simulink model "No5_QuadcopterAltitudeControl"  (R2022a)
settings: Solver=FixedStepDiscrete  StartTime=0.0  StopTime=inf  RelTol=1e-3  EnableMultiTasking=on
undefined symbols (not defined in the file): dev, DiscIntNeverNeededParam, Main, pwm_output0
libraries: simulink x1, px4lib x1, px4uORBlib x1
settings Model: ExtModeTrigDuration=10  Creator=liuwhale  LastModifiedBy=liuwhale
settings SolverCC: PositivePriorityOrder=on
settings OptimizationCC: EnhancedBackFolding=on  PassReuseOutputArgsAs=Individual arguments  ZeroExternalMemoryAtStartup=off  ZeroInternalMemoryAtStartup=off  MaxStackSize=64  OptimizeBlockOrder=speed  DifferentSizesBufferReuse=on  OptimizationCustomize=off  EfficientTunableParamExpr=on
settings DebuggingCC: ParameterTunabilityLossMsg=error
settings HardwareCC: ProdBitPerPointer=32  ProdBitPerSizeT=32  ProdBitPerPtrDiffT=32  ProdLargestAtomicInteger=Long  ProdLargestAtomicFloat=Double  ProdWordSize=32  ProdLongLongMode=on  ProdHWDeviceType=ARM Compatible->ARM Cortex
settings SFSimCC: MATLABDynamicMemAlloc=off  SimTargetLang=C++
settings RTWCC: SystemTargetFile=ert.tlc  HardwareBoard=PX4 Host Target  TLCOptions="-aInlineSetEventsForThisBaseRateFcn=TLC_FALSE -aSuppressMultiTaskScheduler=TLC_FALSE  -aRateBasedStepFcn=0"  TemplateMakefile=ert_default_tmf  Toolchain=GNU Tools for PX4 Autopilots  PortableWordSizes=on  TargetLang=C++
settings CodeAppCC: ForceParamTrailComments=on  IgnoreCustomStorageClasses=off  OperatorAnnotations=on  SimulinkDataObjDesc=on  SFDataObjDesc=on  InsertBlockDesc=on
settings ERTTargetCC: ExtModeStaticAlloc=on

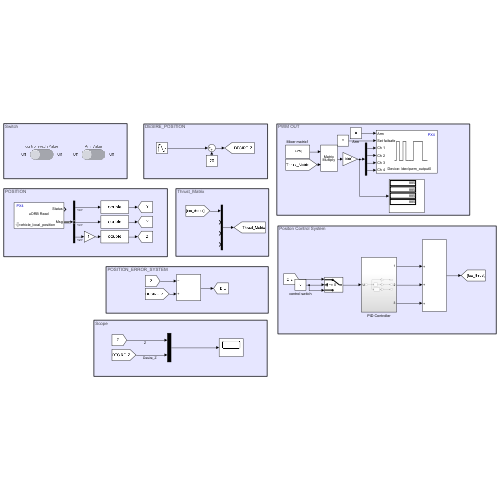
[thumbnail: Simulink's stored preview of the top-level diagram]
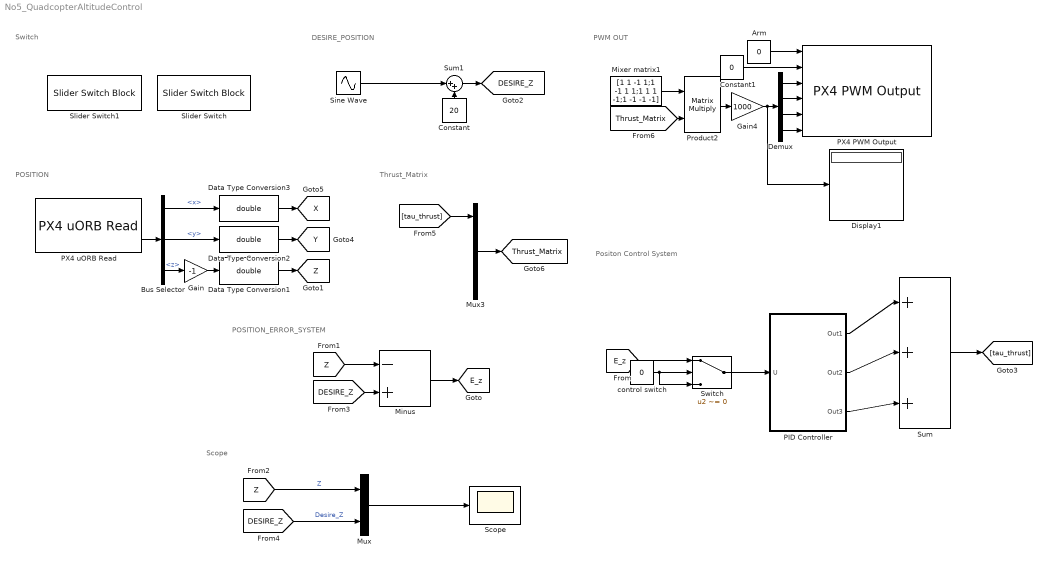
== system No5_QuadcopterAltitudeControl ==
  note: PWM OUT
  note: Scope
  note: Positon Control System
  note: Thrust_Matrix
  note: POSITION_ERROR_SYSTEM
  note: POSITION
  note: DESIRE_POSITION
  note: Switch
  Arm : Constant  Value=0  OutDataTypeStr=boolean
  Bus Selector : BusSelector  OutputSignals=x,y,z
  Constant : Constant  Value=20
  Constant1 : Constant  Value=0  OutDataTypeStr=boolean
  Data Type Conversion1 : DataTypeConversion  OutDataTypeStr=double  SaturateOnIntegerOverflow=off  RndMeth=Floor
  Data Type Conversion2 : DataTypeConversion  OutDataTypeStr=double  SaturateOnIntegerOverflow=off  RndMeth=Floor
  Data Type Conversion3 : DataTypeConversion  OutDataTypeStr=double  SaturateOnIntegerOverflow=off  RndMeth=Floor
  Demux : Demux
  Display1 : Display
  Gain : Gain  Gain=-1
  Gain4 : Gain  Gain=1000  OutDataTypeStr=uint16
  Minus : Sum  Inputs=-+
  Mixer matrix1 : Constant  Value=[1 1 -1 1;1 -1 1 1;1 1 1 -1;1 -1 -1 -1]  OutDataTypeStr=Inherit: Inherit via back propagation
  Mux : Mux  Inputs=2
  Mux3 : Mux
  PID Controller : Subsystem
  PX4 PWM Output : px4lib/PX4 PWM Output  pwmDevice=Main (/dev/pwm_output0)  pwmChannel1_=on  pwmChannel2_=on  pwmChannel3_=on  pwmChannel4_=on  pwmChannel5_=off  pwmChannel6_=off  pwmChannel7_=off  pwmChannel8_=off  forceTerminateFailsafe=off  outputErrorStatus=off
      settings: SourceProductBaseCode=PX4AUTOPILOTS
  PX4 uORB Read : px4uORBlib/PX4 uORB Read  uORBTopic=vehicle_local_position  selectInstance=vehicle_local_position  SampleTime=0.001  BlockingMode=off  BlockTimeout=1e-3
      settings: SourceProductBaseCode=PX4AUTOPILOTS
  Product2 : Product  Multiplication=Matrix(*)  RndMeth=Zero
  Scope : Scope
  Sine Wave : Sin  Amplitude=20  SampleTime=0
  Slider Switch : SliderSwitchBlock
      settings: Values={{'Off', 'On'}, [0 1]}
  Slider Switch1 : SliderSwitchBlock
      settings: Values={{'Off', 'On'}, [0 1]}
  Sum : Sum  Inputs=|+++
  Sum1 : Sum  Inputs=|++
  Switch : Switch  Criteria=u2 ~= 0  SaturateOnIntegerOverflow=off  InputSameDT=off
  control switch : Constant  Value=0
  tag scope: DESIRE_Z=global, E_z=global, Thrust_Matrix=global, X=global, Y=global, Z=global
  wires:
  Arm/1 -> PX4 PWM Output/1
  Constant1/1 -> PX4 PWM Output/2
  Mixer matrix1/1 -> Product2/1
  Product2/1 -> Gain4/1
  Demux/1 -> PX4 PWM Output/3
  Demux/2 -> PX4 PWM Output/4
  Demux/3 -> PX4 PWM Output/5
  Demux/4 -> PX4 PWM Output/6
  Gain4/1 -> Display1/1, Demux/1
  Minus/1 -> [E_z]
  Bus Selector/3 -> Gain/1  "<z>"
  PX4 uORB Read/2 -> Bus Selector/1
  Gain/1 -> Data Type Conversion1/1
  [DESIRE_Z] -> Minus/2
  Mux/1 -> Scope/1
  [Z] -> Mux/1  "Z"
  [DESIRE_Z] -> Mux/2  "Desire_Z"
  [Z] -> Minus/1
  Data Type Conversion1/1 -> [Z]
  Sum1/1 -> [DESIRE_Z]
  Sine Wave/1 -> Sum1/1
  Constant/1 -> Sum1/2
  control switch/1 -> Switch/3, Switch/2
  [E_z] -> Switch/1
  Sum/1 -> [tau_thrust]
  [tau_thrust] -> Mux3/1
  Mux3/1 -> [Thrust_Matrix]
  Data Type Conversion2/1 -> [Y]
  Bus Selector/2 -> Data Type Conversion2/1  "<y>"
  Data Type Conversion3/1 -> [X]
  Bus Selector/1 -> Data Type Conversion3/1  "<x>"
  [Thrust_Matrix] -> Product2/2
  Switch/1 -> PID Controller/1(U)
  PID Controller/1(Out1) -> Sum/1
  PID Controller/2(Out2) -> Sum/2
  PID Controller/3(Out3) -> Sum/3

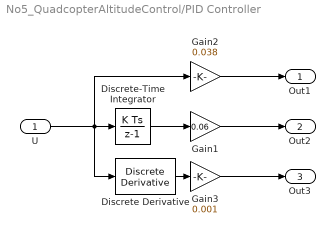
== system No5_QuadcopterAltitudeControl/PID Controller ==
  U : Inport
  Discrete Derivative : simulink/Discrete/Discrete Derivative  gainval=1.0  ICPrevScaledInput=0.0  OutMin=[]  OutMax=[]  OutDataType=fixdt(1, 16)  OutScaling=2^-10  DoSatur=off
  Discrete-Time Integrator : DiscreteIntegrator  SampleTime=-1  ICPrevOutput=DiscIntNeverNeededParam  ICPrevScaledInput=DiscIntNeverNeededParam
  Gain1 : Gain  Gain=0.06
  Gain2 : Gain  Gain=0.038
  Gain3 : Gain  Gain=0.001
  Out1 : Outport
  Out2 : Outport  Port=2
  Out3 : Outport  Port=3
  wires:
  Discrete Derivative/1 -> Gain3/1
  U/1 -> Gain2/1, Discrete-Time Integrator/1, Discrete Derivative/1
  Gain3/1 -> Out3/1
  Gain1/1 -> Out2/1
  Discrete-Time Integrator/1 -> Gain1/1
  Gain2/1 -> Out1/1
